simulink model "DetectBrakeTime"  (Simulink 7.0)
settings: Solver=FixedStepDiscrete  StartTime=0.0  StopTime=inf  RelTol=1e-3
libraries: canoelib x6, simulink x3
settings Model: Creator=visjf  LastModifiedBy=visbma
settings DebuggingCC: MultiTaskCondExecSysMsg=none
settings HardwareCC: TargetHWDeviceType=32-bit Generic
settings RTWCC: SystemTargetFile=cn.tlc  TemplateMakefile=cn_msdll.tmf  Description=Vector CANoe Real-Time Target DLL (Visual C/C++ Project Makefile)  ProcessScript=cn_make_rtw_hook  IncludeERTFirstTime=on
settings STFCustomTargetCC: TargetFcnLib=ansi_tfl_tmw.mat  GenFloatMathFcnCalls=ANSI_C  ModelReferenceCompliant=off  MatFileLogging=on  SystemTargetFile=cn.tlc
settings GRTTargetCC: TargetFcnLib=ansi_tfl_tmw.mat  ModelReferenceCompliant=off  CompOptLevelCompliant=off  ExtModeMexFile=noextcomm  RTWCAPISignals=on  RTWCAPIParams=on
settings CustomProperty: DataType=string  Value=..\..\Exec32

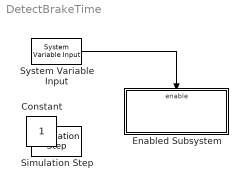
== system DetectBrakeTime ==
  Enabled Subsystem : Subsystem  TreatAsAtomicUnit=on
  Simulation Step : canoelib/CANoe I//O/Simulation Step  SystemSampleTime=-1  mode=Synchronized
      settings: AttributesFormatString=%<mode>
  System Variable Input : canoelib/CANoe I//O/System Variable Input  SystemSampleTime=-1  nsName=Control  sysVarName=brakeActive  arrayIndex=-1  editSampleTime=0
      settings: AttributesFormatString=%<nsName>::%<sysVarName>
  Constant : Constant  IOType=siggen
  wires:
  System Variable Input/1 -> Enabled Subsystem/Enable

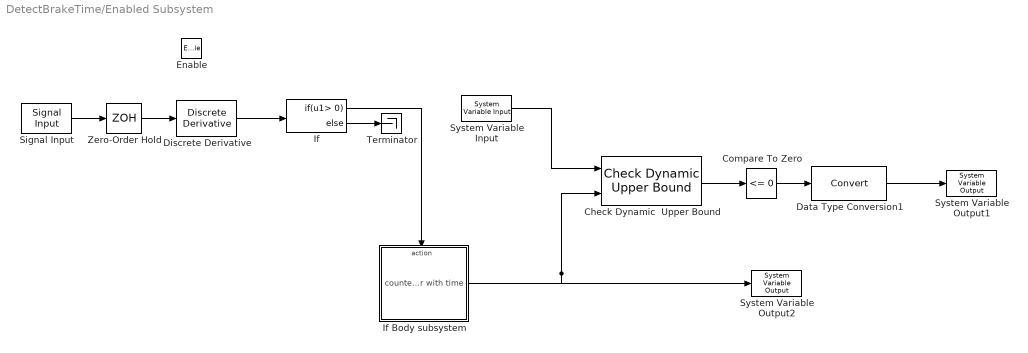
== system DetectBrakeTime/Enabled Subsystem ==
  Enable : EnablePort  StatesWhenEnabling=reset
  Check Dynamic  Upper Bound : simulink/Model Verification/Check Dynamic  Upper Bound  Description=sig < max  SystemSampleTime=-1  enabled=on  stopWhenAssertionFail=off  export=on  icon=graphic
  Compare To Zero : simulink/Logic and Bit Operations/Compare To Zero  SystemSampleTime=-1  relop=<=  LogicOutDataTypeMode=uint8  ZeroCross=off
  Data Type Conversion1 : DataTypeConversion
  Discrete Derivative : simulink/Discrete/Discrete Derivative  SystemSampleTime=-1  gainval=1  ICPrevScaledInput=0.0  OutMin=[]  OutMax=[]  OutDataType=sfix(16)  OutScaling=2^-10  DoSatur=off
  If : If  IfExpression=u1> 0
  If Body subsystem : Subsystem  TreatAsAtomicUnit=on
  Signal Input : canoelib/CANoe I//O/Signal Input  SystemSampleTime=-1  dbName=""  nodeName=""  msgName=""  sigName=xF  editSampleTime=0  rawValue=off
      settings: AttributesFormatString=%<sigName>
  System Variable Input : canoelib/CANoe I//O/System Variable Input  SystemSampleTime=-1  nsName=MatlabIO  sysVarName=SetPointBrakeTime  arrayIndex=-1  editSampleTime=0
      settings: AttributesFormatString=%<nsName>::%<sysVarName>
  System Variable Output1 : canoelib/CANoe I//O/System Variable Output  SystemSampleTime=-1  nsName=MatlabIO  sysVarName=BrakeTimeVerdict  arrayIndex=-1
      settings: AttributesFormatString=%<nsName>::%<sysVarName>
  System Variable Output2 : canoelib/CANoe I//O/System Variable Output  SystemSampleTime=-1  nsName=MatlabIO  sysVarName=BrakeTime  arrayIndex=-1
      settings: AttributesFormatString=%<nsName>::%<sysVarName>
  Terminator : Terminator
  Zero-Order Hold : ZeroOrderHold
  wires:
  Signal Input/1 -> Zero-Order Hold/1
  Zero-Order Hold/1 -> Discrete Derivative/1
  Discrete Derivative/1 -> If/1
  If/1 -> If Body subsystem/Action
  If Body subsystem/1(counter with time) -> Check Dynamic  Upper Bound/2, System Variable Output2/1
  If/2 -> Terminator/1
  System Variable Input/1 -> Check Dynamic  Upper Bound/1
  Compare To Zero/1 -> Data Type Conversion1/1
  Check Dynamic  Upper Bound/1 -> Compare To Zero/1
  Data Type Conversion1/1 -> System Variable Output1/1

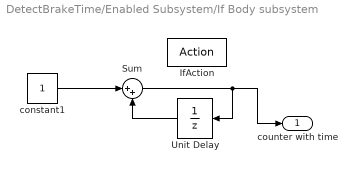
== system DetectBrakeTime/Enabled Subsystem/If Body subsystem ==
  IfAction : ActionPort  InitializeStates=reset  ActionType=then
  Sum : Sum  Inputs=|++  SaturateOnIntegerOverflow=on  InputSameDT=on
  Unit Delay : UnitDelay  Orientation=left
  constant1 : Constant
  counter with time : Outport
  wires:
  Unit Delay/1 -> Sum/2
  constant1/1 -> Sum/1
  Sum/1 -> Unit Delay/1, counter with time/1
